simulink model "sampleDesignR2022b"  (R2024a)
settings: Solver=FixedStepAuto  StartTime=0.0  StopTime=tend  FixedStep=tstep  RelTol=1e-3
settings Model: Creator=Evandson  LastModifiedBy=Evandson
settings DataIOCC: ExternalInput=[t,u]  LoadExternalInput=on  SaveFormat=StructureWithTime

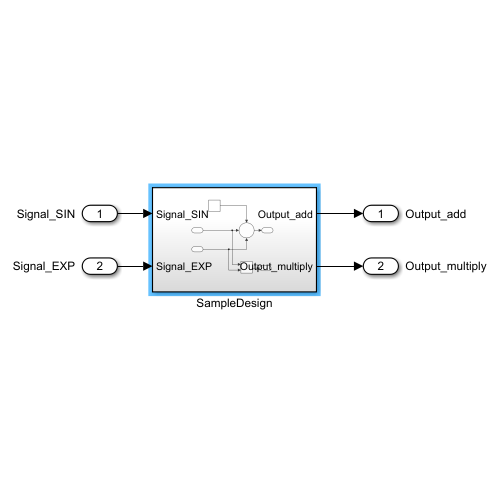
[thumbnail: Simulink's stored preview of the top-level diagram]
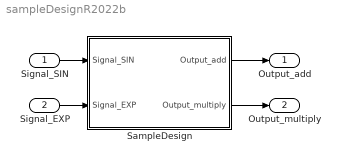
== system sampleDesignR2022b ==
  Signal_SIN : Inport
  Signal_EXP : Inport  Port=2
  SampleDesign : Subsystem
  Output_add : Outport
  Output_multiply : Outport  Port=2
  wires:
  Signal_SIN/1 -> SampleDesign/1(Signal_SIN)
  Signal_EXP/1 -> SampleDesign/2(Signal_EXP)
  SampleDesign/1(Output_add) -> Output_add/1
  SampleDesign/2(Output_multiply) -> Output_multiply/1

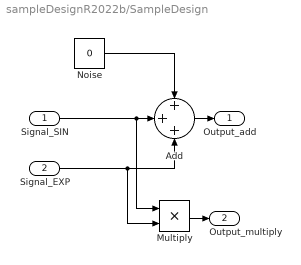
== system sampleDesignR2022b/SampleDesign ==
  Signal_SIN : Inport
  Signal_EXP : Inport  Port=2
  Add : Sum  Inputs=+++
  Multiply : Product  Inputs=**
  Noise : Constant  Value=0
  Output_add : Outport
  Output_multiply : Outport  Port=2
  wires:
  Noise/1 -> Add/1
  Signal_EXP/1 -> Multiply/2, Add/3
  Signal_SIN/1 -> Multiply/1, Add/2
  Multiply/1 -> Output_multiply/1
  Add/1 -> Output_add/1
